simulink model "CubaModelComp"  (R2014a)
settings: Solver=ode3  StartTime=0.0  StopTime=15  FixedStep=0.001  RelTol=1e-3
values from neighbouring files (symbols this model uses):
  C_b = 1.02e-3    (= 0.00102)    [calculateH.m]
  C_w = 0.05e-3    (= 5e-05)    [calculateH.m]
  g = 9.81    [calculateH.m]    (also in initSimulink.m)
  K_D = 2.0107    [initSimulink.m]
  K_I = 5    [initSimulink.m]
  K_P = 3.9208    [initSimulink.m]
  l = 0.085    [calculateH.m]
  l_b = 0.075    [calculateH.m]
  m_b = 0.419    [calculateH.m]
  m_w = 0.204    [calculateH.m]
  O_G_A = O_b_A + m_w * l^2    (= 0.0048139)    [calculateH.m]    (also in initSimulink.m = O_b_A + m_R * l_AB^2)
  O_w_B = 0.57e-3    (= 0.00057)    [calculateH.m]
  phi_b0 = degtorad(0)    [calculateH.m]
  phi_b__d0 = degtorad(0)    [calculateH.m]
  phi_w0 = degtorad(0)    [calculateH.m]
  phi_w__d0 = degtorad(0)    [calculateH.m]
settings Model: CovModelRefEnable=off  CovSFcnEnable=on  Creator=michael  LastModifiedBy=michael
settings DataIOCC: LimitDataPoints=off  SaveFormat=StructureWithTime
settings DebuggingCC: MergeDetectMultiDrivingBlocksExec=error  SolverPrmCheckMsg=none  FrameProcessingCompatibilityMsg=error
settings HardwareCC: ProdBitPerPointer=64  ProdLargestAtomicFloat=Float  ProdIntDivRoundTo=Zero  ProdEndianess=LittleEndian  ProdHWDeviceType=Specified
settings ModelReferenceCC: PropagateSignalLabelsOutOfModel=on

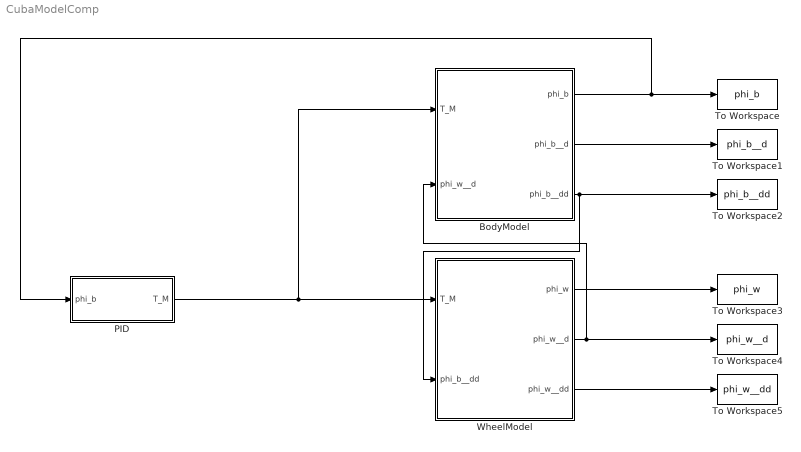
== system CubaModelComp ==
  BodyModel : Subsystem
  PID : Subsystem
  To Workspace : ToWorkspace  VariableName=phi_b  SampleTime=-1
  To Workspace1 : ToWorkspace  VariableName=phi_b__d  SampleTime=-1
  To Workspace2 : ToWorkspace  VariableName=phi_b__dd  SampleTime=-1
  To Workspace3 : ToWorkspace  VariableName=phi_w  SampleTime=-1
  To Workspace4 : ToWorkspace  VariableName=phi_w__d  SampleTime=-1
  To Workspace5 : ToWorkspace  VariableName=phi_w__dd  SampleTime=-1
  WheelModel : Subsystem
  wires:
  WheelModel/2(phi_w__d) -> To Workspace4/1, BodyModel/2(phi_w__d)
  BodyModel/3(phi_b__dd) -> To Workspace2/1, WheelModel/2(phi_b__dd)
  BodyModel/1(phi_b) -> PID/1(phi_b), To Workspace/1
  BodyModel/2(phi_b__d) -> To Workspace1/1
  WheelModel/1(phi_w) -> To Workspace3/1
  WheelModel/3(phi_w__dd) -> To Workspace5/1
  PID/1(T_M) -> BodyModel/1(T_M), WheelModel/1(T_M)

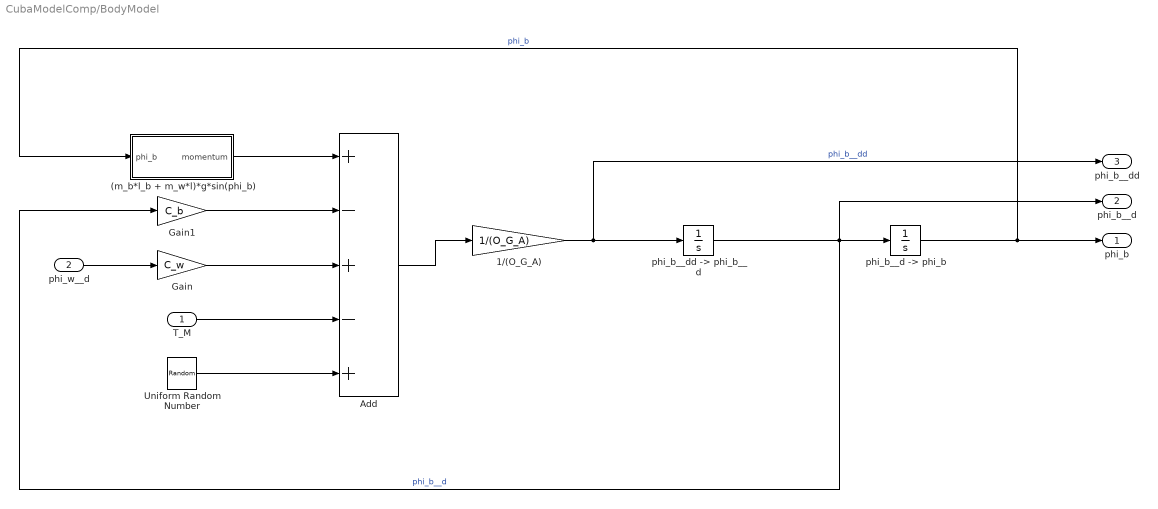
== system CubaModelComp/BodyModel ==
  T_M : Inport
  phi_w__d : Inport  Port=2
  (m_b*l_b + m_w*l)*g*sin(phi_b) : Subsystem
  1/(O_G_A) : Gain  Gain=1/(O_G_A)
  Add : Sum  Inputs=+-+-+
  Gain : Gain  Gain=C_w
  Gain1 : Gain  Gain=C_b
  Uniform Random Number : UniformRandomNumber  Minimum=-0.01  Maximum=0.01  SampleTime=0.001
  "phi_b__d -> phi_b" : Integrator  InitialCondition=phi_b0
  "phi_b__dd -> phi_b__d" : Integrator  InitialCondition=phi_b__d0
  phi_b : Outport
  phi_b__d : Outport  Port=2
  phi_b__dd : Outport  Port=3
  wires:
  T_M/1 -> Add/4
  Gain/1 -> Add/3
  Gain1/1 -> Add/2
  (m_b*l_b + m_w*l)*g*sin(phi_b)/1(momentum) -> Add/1
  phi_w__d/1 -> Gain/1
  Add/1 -> 1/(O_G_A)/1
  1/(O_G_A)/1 -> phi_b__dd/1, "phi_b__dd -> phi_b__d"/1  "phi_b__dd"
  "phi_b__dd -> phi_b__d"/1 -> Gain1/1, phi_b__d/1, "phi_b__d -> phi_b"/1  "phi_b__d"
  "phi_b__d -> phi_b"/1 -> phi_b/1, (m_b*l_b + m_w*l)*g*sin(phi_b)/1(phi_b)  "phi_b"
  Uniform Random Number/1 -> Add/5

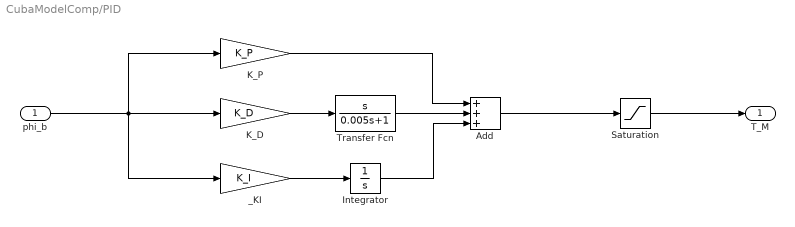
== system CubaModelComp/PID ==
  phi_b : Inport
  Add : Sum  Inputs=+++
  Integrator : Integrator
  K_D : Gain  Gain=K_D
  K_P : Gain  Gain=K_P
  Saturation : Saturate  UpperLimit=0.1  LowerLimit=-0.1
  Transfer Fcn : TransferFcn  Numerator=[1 0]  Denominator=[0.005 1]
  _KI : Gain  Gain=K_I
  T_M : Outport
  wires:
  phi_b/1 -> _KI/1, K_P/1, K_D/1
  _KI/1 -> Integrator/1
  Add/1 -> Saturation/1
  K_D/1 -> Transfer Fcn/1
  Integrator/1 -> Add/3
  K_P/1 -> Add/1
  Transfer Fcn/1 -> Add/2
  Saturation/1 -> T_M/1

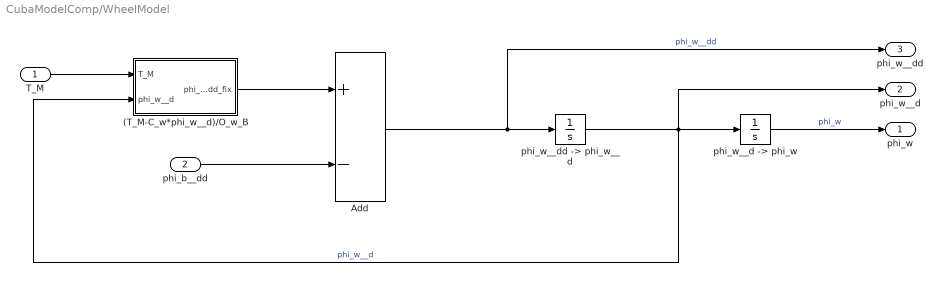
== system CubaModelComp/WheelModel ==
  T_M : Inport
  phi_b__dd : Inport  Port=2
  (T_M-C_w*phi_w__d)/O_w_B : Subsystem
  Add : Sum  Inputs=+-
  "phi_w__d -> phi_w" : Integrator  InitialCondition=phi_w0
  "phi_w__dd -> phi_w__d" : Integrator  InitialCondition=phi_w__d0
  phi_w : Outport
  phi_w__d : Outport  Port=2
  phi_w__dd : Outport  Port=3
  wires:
  phi_b__dd/1 -> Add/2
  Add/1 -> phi_w__dd/1, "phi_w__dd -> phi_w__d"/1  "phi_w__dd"
  "phi_w__dd -> phi_w__d"/1 -> phi_w__d/1, (T_M-C_w*phi_w__d)/O_w_B/2(phi_w__d), "phi_w__d -> phi_w"/1  "phi_w__d"
  (T_M-C_w*phi_w__d)/O_w_B/1(phi_w__dd_fix) -> Add/1
  T_M/1 -> (T_M-C_w*phi_w__d)/O_w_B/1(T_M)
  "phi_w__d -> phi_w"/1 -> phi_w/1  "phi_w"

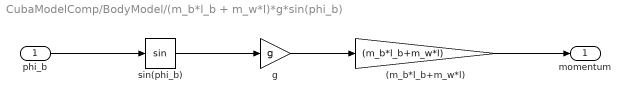
== system CubaModelComp/BodyModel/(m_b*l_b + m_w*l)*g*sin(phi_b) ==
  phi_b : Inport
  (m_b*l_b+m_w*l) : Gain  Gain=(m_b*l_b+m_w*l)
  g : Gain  Gain=g
  sin(phi_b) : Trigonometry
  momentum : Outport
  wires:
  sin(phi_b)/1 -> g/1
  phi_b/1 -> sin(phi_b)/1
  g/1 -> (m_b*l_b+m_w*l)/1
  (m_b*l_b+m_w*l)/1 -> momentum/1

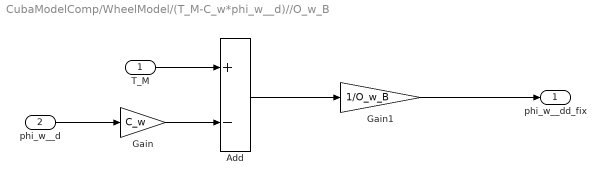
== system CubaModelComp/WheelModel/(T_M-C_w*phi_w__d)//O_w_B ==
  T_M : Inport
  phi_w__d : Inport  Port=2
  Add : Sum  Inputs=+-
  Gain : Gain  Gain=C_w
  Gain1 : Gain  Gain=1/O_w_B
  phi_w__dd_fix : Outport
  wires:
  T_M/1 -> Add/1
  phi_w__d/1 -> Gain/1
  Gain/1 -> Add/2
  Add/1 -> Gain1/1
  Gain1/1 -> phi_w__dd_fix/1
